simulink model "Modell"  (R2023a)
settings: Solver=FixedStepDiscrete  StartTime=0.0  StopTime=10  FixedStep=1/30  RelTol=1e-3
undefined symbols (not defined in the file or in its folder): dsys, K, L, V, x0, x0_hat
settings Model: Creator=Legenden-PC  LastModifiedBy=Legenden-PC
settings OptimizationCC: ReuseModelBlockBuffer=off

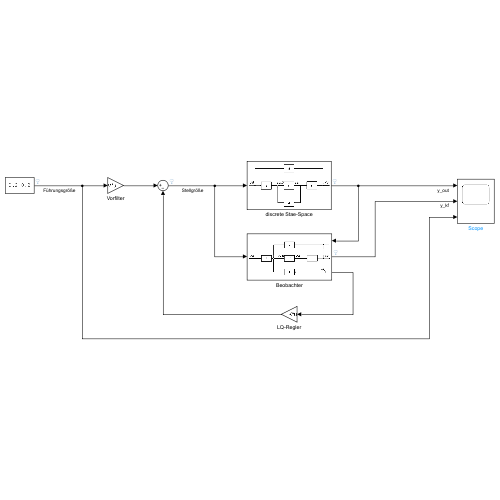
[thumbnail: Simulink's stored preview of the top-level diagram]
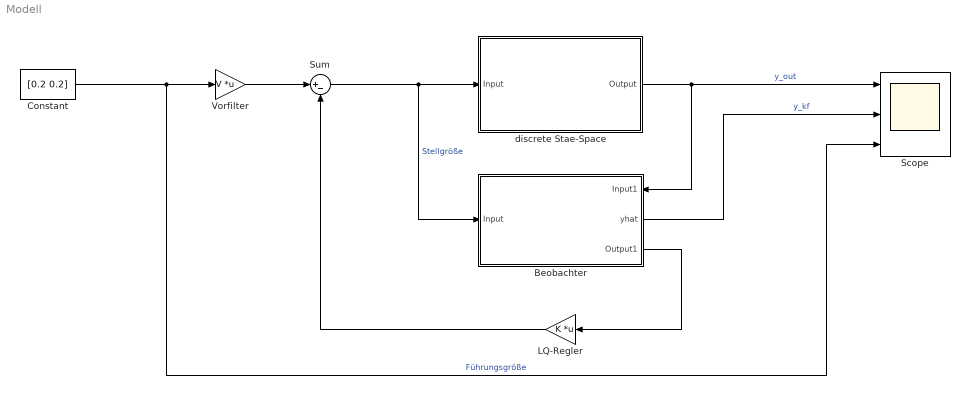
== system Modell ==
  Beobachter : Subsystem
      settings: PortSchema="{\"entries\":[{\"content\":{\"sides\":[{\"content\":{\"connectorIds\":[\"In1\"]},\"type\":\"ConnectorPlacement.EquallySpacedRectSide\",\"uuid\":\"7e5694c5-51f3-4613-b5c8-acc747c9826e\"},{\"content\":{\"connectorIds\":[\"In2\",\"Out1\",\"Out2\"],\"side\":\"RIGHT\"},\"type\":\"ConnectorPlacement.EquallySpacedRectSide\",\"uuid\":\"58036581-f4bf-4920-a29f-01b8659c3d69\"},{\"content\":{\"side\":\"TOP\"},\"type\":\"ConnectorPlacement.EquallySpacedRectSide\",\"uuid\":\"44b743f9-1d96-4ea6-8e40-824e89431d7c\"}]},\"type\":\"ConnectorPlacement.EquallySpacedConnector\",\"uuid\":\"fe3e5cc9-c08e-4053-bf0f-ee9da84c1419\"}],\"packageUris\":[\"http://schema.mathworks.com/mf0/Connector/R2020b\"],\"version\":\"1.0\"}"
      mask Display: image('$imagefile'); % Use "Edit Image" on toolstrip to change.
  Constant : Constant  Value=[0.2 0.2]
  LQ-Regler : Gain  Gain=K  Multiplication=Matrix(K*u)
  Scope : Scope  NumInputPorts=3
  Sum : Sum  Inputs=|+-
  Vorfilter : Gain  Gain=V  Multiplication=Matrix(K*u)
  discrete Stae-Space : Subsystem
      mask Display: image('$imagefile'); % Use "Edit Image" on toolstrip to change.
  wires:
  discrete Stae-Space/1(Output) -> Scope/1, Beobachter/2(Input1)  "y_out"
  Beobachter/2(Output1) -> LQ-Regler/1
  Sum/1 -> discrete Stae-Space/1(Input), Beobachter/1(Input)  "Stellgröße"
  LQ-Regler/1 -> Sum/2
  Vorfilter/1 -> Sum/1
  Constant/1 -> Vorfilter/1, Scope/3  "Führungsgröße"
  Beobachter/1(yhat) -> Scope/2  "y_kf"

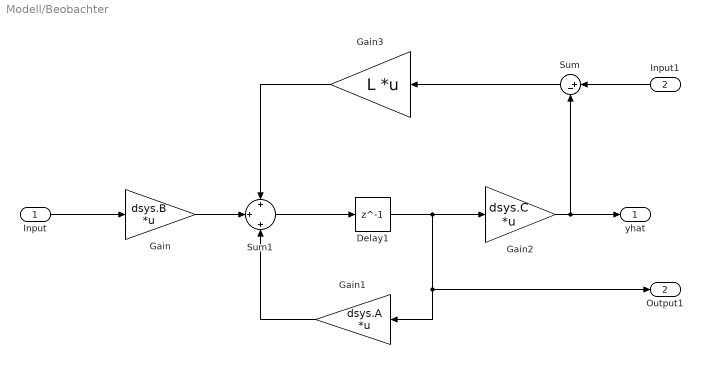
== system Modell/Beobachter ==
  Input : Inport
  Input1 : Inport  Port=2
  Delay1 : Delay  DelayLength=1  InitialCondition=x0_hat
  Gain : Gain  Gain=dsys.B  Multiplication=Matrix(K*u)
  Gain1 : Gain  Gain=dsys.A  Multiplication=Matrix(K*u)
  Gain2 : Gain  Gain=dsys.C  Multiplication=Matrix(K*u)
  Gain3 : Gain  Gain=L  Multiplication=Matrix(K*u)
  Sum : Sum  Inputs=|+-
  Sum1 : Sum  Inputs=+|+|+
  yhat : Outport
  Output1 : Outport  Port=2
  wires:
  Input/1 -> Gain/1
  Gain/1 -> Sum1/2
  Sum1/1 -> Delay1/1
  Delay1/1 -> Gain1/1, Output1/1, Gain2/1
  Gain1/1 -> Sum1/3
  Gain3/1 -> Sum1/1
  Gain2/1 -> yhat/1, Sum/2
  Sum/1 -> Gain3/1
  Input1/1 -> Sum/1

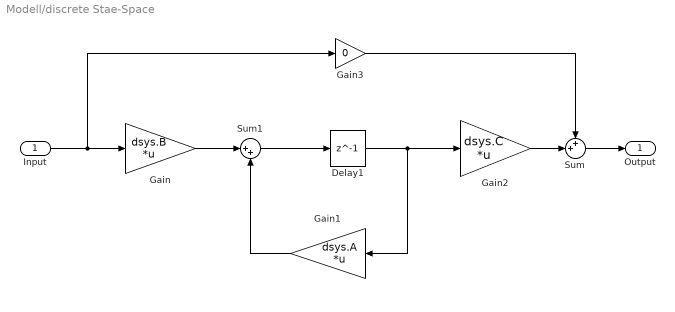
== system Modell/discrete Stae-Space ==
  Input : Inport
  Delay1 : Delay  DelayLength=1  InitialCondition=x0
  Gain : Gain  Gain=dsys.B  Multiplication=Matrix(K*u)
  Gain1 : Gain  Gain=dsys.A  Multiplication=Matrix(K*u)
  Gain2 : Gain  Gain=dsys.C  Multiplication=Matrix(K*u)
  Gain3 : Gain  Gain=0
  Sum : Sum  Inputs=++|
  Sum1 : Sum  Inputs=|++
  Output : Outport
  wires:
  Input/1 -> Gain3/1, Gain/1
  Gain/1 -> Sum1/1
  Sum1/1 -> Delay1/1
  Delay1/1 -> Gain1/1, Gain2/1
  Gain1/1 -> Sum1/2
  Gain2/1 -> Sum/2
  Gain3/1 -> Sum/1
  Sum/1 -> Output/1
